simulink model "lqr_cartpend_sim"  (R2015b)
settings: Solver=VariableStepAuto  StartTime=0.0  StopTime=50.0  RelTol=1e-3
values from neighbouring files (symbols this model uses):
  K = lqr(A,B,Q,R)    [lqg_simulinkINIT.m]    (also in lqg_simulinkINITBOOK.m)
settings Model: Creator=sbrunton  LastModifiedBy=sbrunton

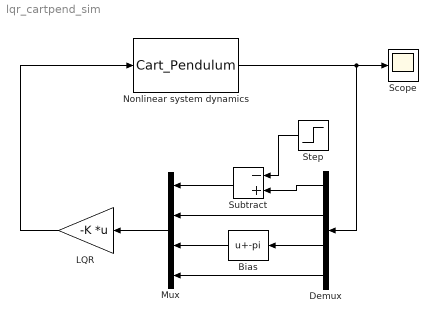
== system lqr_cartpend_sim ==
  Bias : Bias  Bias=-pi
  Demux : Demux
  LQR : Gain  Gain=-K  Multiplication=Matrix(K*u) (u vector)
  Mux : Mux
  Nonlinear system dynamics : S-Function  InitFcn=try, set_param(gcb,'FunctionName','Cart_Pendulum'), end  FunctionName=Cart_Pendulum  SFunctionModules=cartpend_sim_wrapper  SFunctionDeploymentMode=off  EnableBusSupport=off  mask(S-Function Builder){}
      mask help: Simulink:masks:SFunctionBuilder_MD
      mask init:
      | val = [[.9  0.75 0.75 1 1 .9 .9 1]',[1 1 0.75 0.75 .9 .9 1 .9]'];try , sys = get_param(gcb,'SfunBuilderFcnName');if isempty(sys), sys = get_param(gcb,'FunctionName'); end,catch, sys = get_param(gcb,'FunctionName'); end
      settings: CopyFcn=set_param(gcbh,'LinkStatus','none')  PreSaveFcn=try, set_param(gcb,'FunctionName','Cart_Pendulum'), end  OpenFcn=sfunctionwizard(gcbh)
      mask Display: plot(val(:,1),val(:,2)),disp(sys), port_label('input',1,'u'), port_label('output',1,'x')
  Scope : Scope
  Step : Step  Time=10  SampleTime=0
  Subtract : Sum  Inputs=-+
  wires:
  LQR/1 -> Nonlinear system dynamics/1
  Nonlinear system dynamics/1 -> Demux/1, Scope/1
  Demux/2 -> Mux/2
  Demux/4 -> Mux/4
  Demux/3 -> Bias/1
  Bias/1 -> Mux/3
  Mux/1 -> LQR/1
  Subtract/1 -> Mux/1
  Step/1 -> Subtract/1
  Demux/1 -> Subtract/2
